simulink model "stateflow_ex2"  (R2023a)
settings: Solver=FixedStepAuto  StartTime=0.0  StopTime=1  FixedStep=0.1  RelTol=1e-3
settings Model: Creator=ArriGE66  LastModifiedBy=ArriGE66
settings ModelReferenceCC: EnableRefExpFcnMdlSchedulingChecks=on

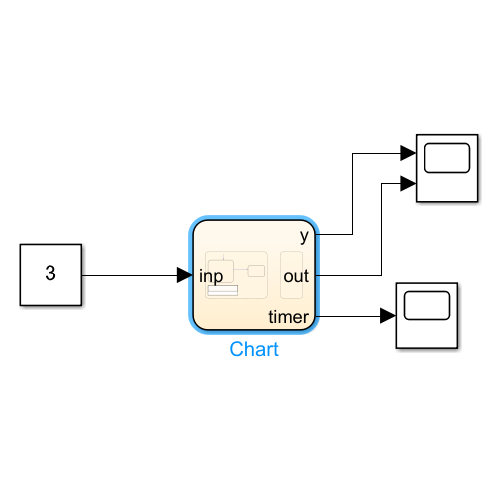
[thumbnail: Simulink's stored preview of the top-level diagram]
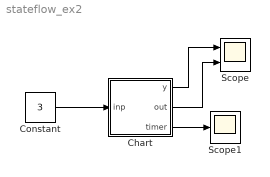
== system stateflow_ex2 ==
  Chart : Stateflow chart  TreatAsAtomicUnit=on
  Constant : Constant  Value=3
  Scope : Scope  NumInputPorts=2
  Scope1 : Scope
  wires:
  Chart/1(y) -> Scope/1
  Chart/2(out) -> Scope/2
  Constant/1 -> Chart/1(inp)
  Chart/3(timer) -> Scope1/1

== stateflow chart stateflow_ex2/Chart ==
  state super_state [parallel]
    settings: executionOrder=1
    state init_state
      en:
      x=0; y=x; out=-1;
      du:
      x=x+1; y=x;
      out=multiply(y,inp);
      ex:
      y=-1;
    state stateA
      %y=-3;
      out=0;
    (default) -> init_state
    init_state -> stateA : [x>5]
  state timer [parallel]
    en: timer=0;
    du: timer=timer+1;
    settings: executionOrder=2
  data: var1 function_input; var2 function_input; var3 function_output; y output; x local; out output; inp input; timer output
  function var3 =multiply(var1,var2):
    | function var3 =multiply(var1,var2)
    |  
    | var3=var1*var2;
